simulink model "PickAndPlace_WithSelector"  (R2022b)
settings: Solver=ode4  StartTime=0.0  StopTime=Inf  FixedStep=1/500  RelTol=1e-3
InitFcn:
  | home = [0.45; 0; 0.49];
  | pick = [0.66; 0; 0.3];
  | place = [-0.425; 0.5; 0.35];
  | 
  | waypoints = ...
  | [pick, pick, place, place, home]' ;
undefined symbols (not defined in the file): HIL, pick2, place2, qc_get_step_size, waypoints2
libraries: quarc_library x5
settings Model: ExtModeTrigDuration=10000  Creator=fvranes  LastModifiedBy=user
settings SolverCC: AlgebraicLoopSolver=TrustRegion
settings DataIOCC: ReturnWorkspaceOutputs=off
settings DebuggingCC: UnderspecifiedInitializationDetection=Classic  MergeDetectMultiDrivingBlocksExec=none  UnconnectedInputMsg=warning  UnconnectedOutputMsg=warning  UnconnectedLineMsg=warning  SFMachineParentedDataDiag=warning
settings ModelReferenceCC: EnableRefExpFcnMdlSchedulingChecks=on  PropagateSignalLabelsOutOfModel=off
settings SFSimCC: CustomCodeUndefinedFunction=UseInterfaceOnly

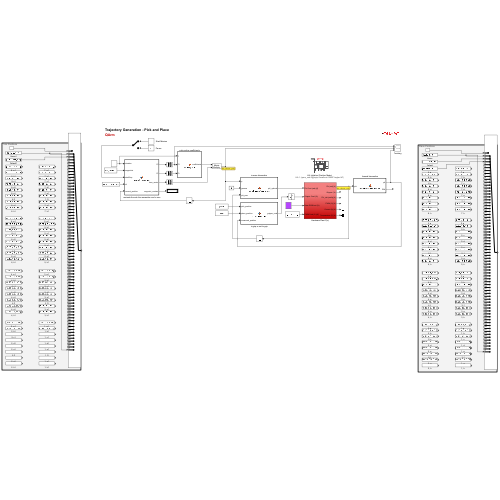
[thumbnail: Simulink's stored preview of the top-level diagram]
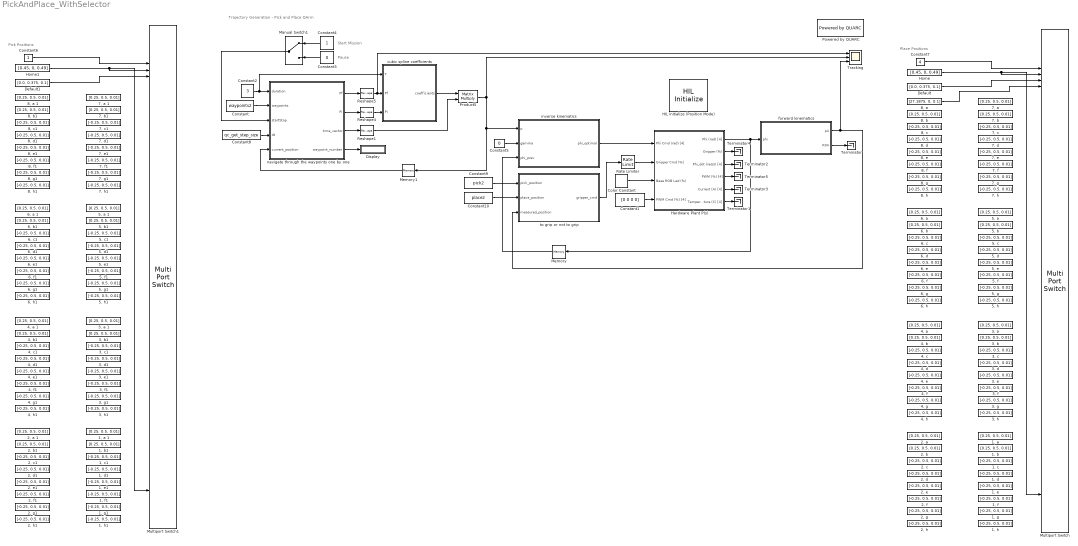
== system PickAndPlace_WithSelector ==
  note: Pause
  note: Start Mission
  note: Trajectory Generation - Pick and Place
      | QArm
  note: Place Positions
  note: Pick Positions
  "1, a " : Constant  Value=[0.25, 0.5, 0.01]
  "1, a 1" : Constant  Value=[0.25, 0.5, 0.01]
  "1, b" : Constant  Value=[0.25, 0.5, 0.01]
  "1, b1" : Constant  Value=[0.25, 0.5, 0.01]
  "1, c" : Constant  Value=[-0.25, 0.5, 0.01]
  "1, c1" : Constant  Value=[-0.25, 0.5, 0.01]
  "1, d" : Constant  Value=[-0.25, 0.5, 0.01]
  "1, d1" : Constant  Value=[-0.25, 0.5, 0.01]
  "1, e" : Constant  Value=[-0.25, 0.5, 0.01]
  "1, e1" : Constant  Value=[-0.25, 0.5, 0.01]
  "1, f" : Constant  Value=[-0.25, 0.5, 0.01]
  "1, f1" : Constant  Value=[-0.25, 0.5, 0.01]
  "1, g" : Constant  Value=[-0.25, 0.5, 0.01]
  "1, g1" : Constant  Value=[-0.25, 0.5, 0.01]
  "1, h" : Constant  Value=[-0.25, 0.5, 0.01]
  "1, h1" : Constant  Value=[-0.25, 0.5, 0.01]
  "2, a " : Constant  Value=[0.25, 0.5, 0.01]
  "2, a 1" : Constant  Value=[0.25, 0.5, 0.01]
  "2, b" : Constant  Value=[0.25, 0.5, 0.01]
  "2, b1" : Constant  Value=[0.25, 0.5, 0.01]
  "2, c" : Constant  Value=[-0.25, 0.5, 0.01]
  "2, c1" : Constant  Value=[-0.25, 0.5, 0.01]
  "2, d" : Constant  Value=[-0.25, 0.5, 0.01]
  "2, d1" : Constant  Value=[-0.25, 0.5, 0.01]
  "2, e" : Constant  Value=[-0.25, 0.5, 0.01]
  "2, e1" : Constant  Value=[-0.25, 0.5, 0.01]
  "2, f" : Constant  Value=[-0.25, 0.5, 0.01]
  "2, f1" : Constant  Value=[-0.25, 0.5, 0.01]
  "2, g" : Constant  Value=[-0.25, 0.5, 0.01]
  "2, g1" : Constant  Value=[-0.25, 0.5, 0.01]
  "2, h" : Constant  Value=[-0.25, 0.5, 0.01]
  "2, h1" : Constant  Value=[-0.25, 0.5, 0.01]
  "3, a " : Constant  Value=[0.25, 0.5, 0.01]
  "3, a 1" : Constant  Value=[0.25, 0.5, 0.01]
  "3, b" : Constant  Value=[0.25, 0.5, 0.01]
  "3, b1" : Constant  Value=[0.25, 0.5, 0.01]
  "3, c" : Constant  Value=[-0.25, 0.5, 0.01]
  "3, c1" : Constant  Value=[-0.25, 0.5, 0.01]
  "3, d" : Constant  Value=[-0.25, 0.5, 0.01]
  "3, d1" : Constant  Value=[-0.25, 0.5, 0.01]
  "3, e" : Constant  Value=[-0.25, 0.5, 0.01]
  "3, e1" : Constant  Value=[-0.25, 0.5, 0.01]
  "3, f" : Constant  Value=[-0.25, 0.5, 0.01]
  "3, f1" : Constant  Value=[-0.25, 0.5, 0.01]
  "3, g" : Constant  Value=[-0.25, 0.5, 0.01]
  "3, g1" : Constant  Value=[-0.25, 0.5, 0.01]
  "3, h" : Constant  Value=[-0.25, 0.5, 0.01]
  "3, h1" : Constant  Value=[-0.25, 0.5, 0.01]
  "4, a " : Constant  Value=[0.25, 0.5, 0.01]
  "4, a 1" : Constant  Value=[0.25, 0.5, 0.01]
  "4, b" : Constant  Value=[0.25, 0.5, 0.01]
  "4, b1" : Constant  Value=[0.25, 0.5, 0.01]
  "4, c" : Constant  Value=[-0.25, 0.5, 0.01]
  "4, c1" : Constant  Value=[-0.25, 0.5, 0.01]
  "4, d" : Constant  Value=[-0.25, 0.5, 0.01]
  "4, d1" : Constant  Value=[-0.25, 0.5, 0.01]
  "4, e" : Constant  Value=[-0.25, 0.5, 0.01]
  "4, e1" : Constant  Value=[-0.25, 0.5, 0.01]
  "4, f" : Constant  Value=[-0.25, 0.5, 0.01]
  "4, f1" : Constant  Value=[-0.25, 0.5, 0.01]
  "4, g" : Constant  Value=[-0.25, 0.5, 0.01]
  "4, g1" : Constant  Value=[-0.25, 0.5, 0.01]
  "4, h" : Constant  Value=[-0.25, 0.5, 0.01]
  "4, h1" : Constant  Value=[-0.25, 0.5, 0.01]
  "5, a " : Constant  Value=[0.25, 0.5, 0.01]
  "5, a 1" : Constant  Value=[0.25, 0.5, 0.01]
  "5, b" : Constant  Value=[0.25, 0.5, 0.01]
  "5, b1" : Constant  Value=[0.25, 0.5, 0.01]
  "5, c" : Constant  Value=[-0.25, 0.5, 0.01]
  "5, c1" : Constant  Value=[-0.25, 0.5, 0.01]
  "5, d" : Constant  Value=[-0.25, 0.5, 0.01]
  "5, d1" : Constant  Value=[-0.25, 0.5, 0.01]
  "5, e" : Constant  Value=[-0.25, 0.5, 0.01]
  "5, e1" : Constant  Value=[-0.25, 0.5, 0.01]
  "5, f" : Constant  Value=[-0.25, 0.5, 0.01]
  "5, f1" : Constant  Value=[-0.25, 0.5, 0.01]
  "5, g" : Constant  Value=[-0.25, 0.5, 0.01]
  "5, g1" : Constant  Value=[-0.25, 0.5, 0.01]
  "5, h" : Constant  Value=[-0.25, 0.5, 0.01]
  "5, h1" : Constant  Value=[-0.25, 0.5, 0.01]
  "6, a " : Constant  Value=[0.25, 0.5, 0.01]
  "6, a 1" : Constant  Value=[0.25, 0.5, 0.01]
  "6, b" : Constant  Value=[0.25, 0.5, 0.01]
  "6, b1" : Constant  Value=[0.25, 0.5, 0.01]
  "6, c" : Constant  Value=[-0.25, 0.5, 0.01]
  "6, c1" : Constant  Value=[-0.25, 0.5, 0.01]
  "6, d" : Constant  Value=[-0.25, 0.5, 0.01]
  "6, d1" : Constant  Value=[-0.25, 0.5, 0.01]
  "6, e" : Constant  Value=[-0.25, 0.5, 0.01]
  "6, e1" : Constant  Value=[-0.25, 0.5, 0.01]
  "6, f" : Constant  Value=[-0.25, 0.5, 0.01]
  "6, f1" : Constant  Value=[-0.25, 0.5, 0.01]
  "6, g" : Constant  Value=[-0.25, 0.5, 0.01]
  "6, g1" : Constant  Value=[-0.25, 0.5, 0.01]
  "6, h" : Constant  Value=[-0.25, 0.5, 0.01]
  "6, h1" : Constant  Value=[-0.25, 0.5, 0.01]
  "7, a " : Constant  Value=[0.25, 0.5, 0.01]
  "7, a 1" : Constant  Value=[0.25, 0.5, 0.01]
  "7, b" : Constant  Value=[0.25, 0.5, 0.01]
  "7, b1" : Constant  Value=[0.25, 0.5, 0.01]
  "7, c" : Constant  Value=[-0.25, 0.5, 0.01]
  "7, c1" : Constant  Value=[-0.25, 0.5, 0.01]
  "7, d" : Constant  Value=[-0.25, 0.5, 0.01]
  "7, d1" : Constant  Value=[-0.25, 0.5, 0.01]
  "7, e" : Constant  Value=[-0.25, 0.5, 0.01]
  "7, e1" : Constant  Value=[-0.25, 0.5, 0.01]
  "7, f" : Constant  Value=[-0.25, 0.5, 0.01]
  "7, f1" : Constant  Value=[-0.25, 0.5, 0.01]
  "7, g" : Constant  Value=[-0.25, 0.5, 0.01]
  "7, g1" : Constant  Value=[-0.25, 0.5, 0.01]
  "7, h" : Constant  Value=[-0.25, 0.5, 0.01]
  "7, h1" : Constant  Value=[-0.25, 0.5, 0.01]
  "8, a " : Constant  Value=[27.1875, 0, 0.1]
  "8, a 1" : Constant  Value=[0.25, 0.5, 0.01]
  "8, b" : Constant  Value=[0.25, 0.5, 0.01]
  "8, b1" : Constant  Value=[0.25, 0.5, 0.01]
  "8, c" : Constant  Value=[-0.25, 0.5, 0.01]
  "8, c1" : Constant  Value=[-0.25, 0.5, 0.01]
  "8, d" : Constant  Value=[-0.25, 0.5, 0.01]
  "8, d1" : Constant  Value=[-0.25, 0.5, 0.01]
  "8, e" : Constant  Value=[-0.25, 0.5, 0.01]
  "8, e1" : Constant  Value=[-0.25, 0.5, 0.01]
  "8, f" : Constant  Value=[-0.25, 0.5, 0.01]
  "8, f1" : Constant  Value=[-0.25, 0.5, 0.01]
  "8, g" : Constant  Value=[-0.25, 0.5, 0.01]
  "8, g1" : Constant  Value=[-0.25, 0.5, 0.01]
  "8, h" : Constant  Value=[-0.25, 0.5, 0.01]
  "8, h1" : Constant  Value=[-0.25, 0.5, 0.01]
  Color Constant : quarc_library/Sources/Signals/Color Constant  color=[0.71765 0.27451 1]
      settings: SourceProductName=QUARC Targets
  Constant : Constant  Value=waypoints2  VectorParams1D=off
  Constant1 : Constant  Value=[0 0 0 0]
  Constant10 : Constant  Value=place2  VectorParams1D=off
  Constant2 : Constant  Value=3
  Constant3 : Constant  Value=0
  Constant4 : Constant
  Constant5 : Constant  Value=0
  Constant6 : Constant
  Constant7 : Constant  Value=4
  Constant8 : Constant  Value=qc_get_step_size
  Constant9 : Constant  Value=pick2
  Default : Constant  Value=[0.0, 0.375, 0.1]
  Default1 : Constant  Value=[0.0, 0.375, 0.1]
  Display : Display
      settings: Decimation=2
  HIL Initialize (Position Mode) : quarc_library/Data Acquisition/Generic/Configuration/HIL Initialize  object_name=HIL-1  board_type=qarm_usb  board_number=0@tcpip://localhost:18900?nagle='off'  board_options=j0_mode=0;j1_mode=0;j2_mode=0;j3_mode=0;gripper_mode=0;  exclusive=off  active=on  hardware_clocks=[0]  clock_modes=[]  initial_clock_frequencies=[]  set_clock_params_at_start=off  set_clock_params_at_switch_in=off  set_clock_frequencies_at_start=off  set_clock_frequencies_at_switch_in=off  analog_input_channels=[5:9]  analog_input_configurations=[]  analog_input_maximums=[]  analog_input_minimums=[]  set_analog_input_params_at_start=off  set_analog_input_params_at_switch_in=off  analog_output_channels=[]  analog_output_maximums=inf  analog_output_minimums=-inf  initial_analog_outputs=[0]  final_analog_outputs=[0]  watchdog_analog_outputs=[]  set_analog_output_params_at_start=off  set_analog_output_params_at_switch_in=off  set_analog_outputs_at_start=off  set_analog_outputs_at_switch_in=off  set_analog_outputs_at_terminate=off  set_analog_outputs_at_switch_out=off  set_analog_outputs_on_watchdog=off  digital_input_channels=[]  digital_output_channels=[]  digital_output_configuration=[]  initial_digital_outputs=[0]  final_digital_outputs=[0]  watchdog_digital_outputs=[0]  set_digital_output_params_at_start=off  set_digital_output_params_at_switch_in=off  set_digital_outputs_at_start=off  set_digital_outputs_at_switch_in=off  set_digital_outputs_at_terminate=off  set_digital_outputs_at_switch_out=off  set_digital_outputs_on_watchdog=off  encoder_channels=[]  quadrature=[]  encoder_filter_frequency=[]  initial_encoder_counts=[]  set_encoder_params_at_start=off  set_encoder_params_at_switch_in=off  set_encoder_counts_at_start=off  set_encoder_counts_at_switch_in=off  pwm_channels=[]  pwm_modes=[]  pwm_frequency=[]  pwm_configuration=[]  pwm_alignment=[]  pwm_polarity=[]  pwm_leading_deadband=[]  pwm_trailing_deadband=[]  initial_pwm_outputs=[]  final_pwm_outputs=[]  watchdog_pwm_outputs=[]  set_pwm_params_at_start=off  set_pwm_params_at_switch_in=off  set_pwm_outputs_at_start=off  set_pwm_outputs_at_switch_in=off  set_pwm_outputs_at_terminate=off  set_pwm_outputs_at_switch_out=off  set_pwm_outputs_on_watchdog=off  other_output_channels=[1000:1004 11000:11003 11005:11007]  initial_other_outputs=[zeros(1,9), ones(1,3)]  final_other_outputs=[zeros(1,9), ones(1,3)]  watchdog_other_outputs=zeros(1,12)  set_other_outputs_at_start=off  set_other_outputs_at_switch_in=off  set_other_outputs_at_terminate=on  set_other_outputs_at_switch_out=off  set_other_outputs_on_watchdog=off
  Hardware Plant P(s) : Subsystem
  Home : Constant  Value=[0.45, 0, 0.49]
  Home1 : Constant  Value=[0.45, 0, 0.49]
  Manual Switch1 : ManualSwitch
  Memory : Memory
  Memory1 : Memory  InitialCondition=[0.45;0;0.49]
  Multiport Switch : MultiPortSwitch  Inputs=67  DataPortForDefault=Additional data port  SaturateOnIntegerOverflow=off  InputSameDT=off
  Multiport Switch1 : MultiPortSwitch  Inputs=67  DataPortForDefault=Additional data port  SaturateOnIntegerOverflow=off  InputSameDT=off
  Powered by QUARC : quarc_library/Logos/Powered by QUARC
  Product5 : Product  Multiplication=Matrix(*)
  Rate Limiter : RateLimiter  SampleTimeMode=inherited
  Reshape1 : Reshape  OutputDimensionality=Column vector (2-D)
  Reshape4 : Reshape  OutputDimensionality=Column vector (2-D)
  Reshape5 : Reshape  OutputDimensionality=Column vector (2-D)
  Terminator{,1..5} (6 alike) : Terminator
  Tracking : Scope  NumInputPorts=3
  cubic spline coefficients : MATLAB Function  TreatAsAtomicUnit=on
  forward kinematics : MATLAB Function  TreatAsAtomicUnit=on
  inverse kinematics : MATLAB Function  TreatAsAtomicUnit=on
  navigate through the waypoints one by one : MATLAB Function  TreatAsAtomicUnit=on
  to grip or not to grip : MATLAB Function  TreatAsAtomicUnit=on
  wires:
  Hardware Plant P(s)/4(PWM (%) [4]) -> Terminator5/1
  Hardware Plant P(s)/3(Phi_dot (rad/s) [4]) -> Terminator2/1
  Reshape1/1 -> Product5/2
  Hardware Plant P(s)/6(Temperature (C) [4]) -> Terminator1/1
  Memory1/1 -> navigate through the waypoints one by one/5(current_position)
  Memory/1 -> inverse kinematics/3(phi_prev)
  Rate Limiter/1 -> Hardware Plant P(s)/2(Gripper Cmd (%))
  Hardware Plant P(s)/5(Current (A) [4]) -> Terminator3/1
  Reshape4/1 -> cubic spline coefficients/3(Pi)
  Constant8/1 -> navigate through the waypoints one by one/4(dt)
  Color Constant/1 -> Hardware Plant P(s)/3(Base RGB Led (%))
  Constant3/1 -> Manual Switch1/2
  Constant1/1 -> Hardware Plant P(s)/4(PWM Cmd (%) [4])
  Manual Switch1/1 -> navigate through the waypoints one by one/3(startStop)
  Reshape5/1 -> Tracking/1, cubic spline coefficients/2(Pf)
  navigate through the waypoints one by one/4(waypoint_number) -> Display/1
  navigate through the waypoints one by one/1(Pf) -> Reshape5/1
  Hardware Plant P(s)/1(Phi (rad) [4]) -> forward kinematics/1(phi), Memory/1
  Constant5/1 -> inverse kinematics/2(gamma)
  Product5/1 -> Memory1/1, inverse kinematics/1(p), Tracking/2
  navigate through the waypoints one by one/2(Pi) -> Reshape4/1
  Constant4/1 -> Manual Switch1/1
  cubic spline coefficients/1(coefficients) -> Product5/1
  Constant2/1 -> cubic spline coefficients/1(T), navigate through the waypoints one by one/1(duration)
  forward kinematics/2(R04) -> Terminator/1
  forward kinematics/1(p4) -> Tracking/3, to grip or not to grip/3(measured_position)
  inverse kinematics/1(phi_optimal) -> Hardware Plant P(s)/1(Phi Cmd (rad) [4])
  to grip or not to grip/1(gripper_cmd) -> Rate Limiter/1
  navigate through the waypoints one by one/3(time_vector) -> Reshape1/1
  Hardware Plant P(s)/2(Gripper (%)) -> Terminator4/1
  Constant7/1 -> Multiport Switch/1
  Home/1 -> Multiport Switch/69, Multiport Switch/2
  Default/1 -> Multiport Switch/3
  Home1/1 -> Multiport Switch1/69, Multiport Switch1/2
  Constant6/1 -> Multiport Switch1/1
  Default1/1 -> Multiport Switch1/3
  "8, a "/1 -> Multiport Switch/4
  Constant10/1 -> to grip or not to grip/2(place_position)
  Constant9/1 -> to grip or not to grip/1(pick_position)
  Constant/1 -> navigate through the waypoints one by one/2(waypoints)

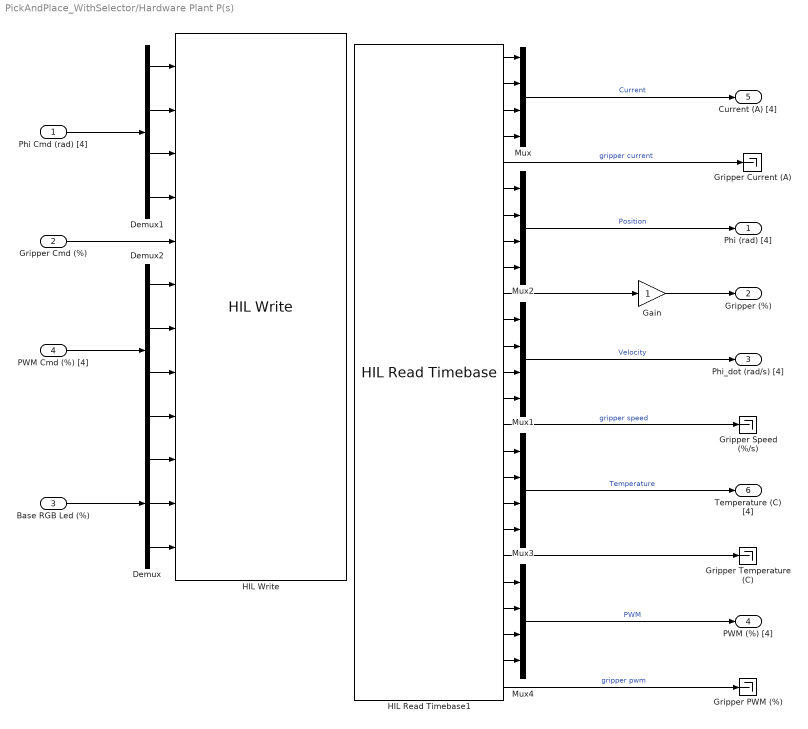
== system PickAndPlace_WithSelector/Hardware Plant P(s) ==
  Phi Cmd (rad) [4] : Inport
  Gripper Cmd (%) : Inport  Port=2
  Base RGB Led (%) : Inport  Port=3
  PWM Cmd (%) [4] : Inport  Port=4
  Demux : Demux  Outputs=3
  Demux1 : Demux
  Demux2 : Demux
  Gain : Gain
  Gripper Current (A) : Terminator
  Gripper PWM (%) : Terminator
  Gripper Speed (%/s) : Terminator
  Gripper Temperature (C) : Terminator
  HIL Read Timebase1 : quarc_library/Data Acquisition/Generic/Timebases/HIL Read Timebase  object_name=HIL-1  clock=0  analog_channels=[5:9]  encoder_channels=[]  digital_channels=[]  other_channels=[1000:1004 3000:3004 10000:10004 11000:11004]  active=on  vector_output=off  data_type_mode=Inherit via back propagation  encoder_data_type=double  digital_data_type=boolean  overflow_mode=Synchronize (for simulated cards only)  samples_in_buffer=1
  HIL Write : quarc_library/Data Acquisition/Generic/Immediate I//O/HIL Write  object_name=HIL-1  analog_channels=[]  pwm_channels=[]  digital_channels=[]  other_channels=[1000:1004 11000:11003 11005:11007]  sample_time=-1  active=on  vector_input=off
  Mux{,1..4} (5 alike) : Mux
  Phi (rad) [4] : Outport  VectorParamsAs1DForOutWhenUnconnected=off
  Gripper (%) : Outport  Port=2  VectorParamsAs1DForOutWhenUnconnected=off
  Phi_dot (rad/s) [4] : Outport  Port=3  VectorParamsAs1DForOutWhenUnconnected=off
  PWM (%) [4] : Outport  Port=4  VectorParamsAs1DForOutWhenUnconnected=off
  Current (A) [4] : Outport  Port=5  VectorParamsAs1DForOutWhenUnconnected=off
  Temperature (C) [4] : Outport  Port=6  VectorParamsAs1DForOutWhenUnconnected=off
  wires:
  HIL Read Timebase1/14 -> Mux1/4
  HIL Read Timebase1/9 -> Mux2/4
  HIL Read Timebase1/6 -> Mux2/1
  HIL Read Timebase1/18 -> Mux3/3
  HIL Read Timebase1/8 -> Mux2/3
  HIL Read Timebase1/12 -> Mux1/2
  HIL Read Timebase1/4 -> Mux/4
  HIL Read Timebase1/7 -> Mux2/2
  HIL Read Timebase1/5 -> Gripper Current (A)/1  "gripper current"
  HIL Read Timebase1/15 -> Gripper Speed (%/s)/1  "gripper speed"
  Demux/3 -> HIL Write/12
  HIL Read Timebase1/3 -> Mux/3
  HIL Read Timebase1/17 -> Mux3/2
  HIL Read Timebase1/16 -> Mux3/1
  HIL Read Timebase1/11 -> Mux1/1
  Demux/1 -> HIL Write/10
  HIL Read Timebase1/19 -> Mux3/4
  Demux/2 -> HIL Write/11
  HIL Read Timebase1/13 -> Mux1/3
  HIL Read Timebase1/2 -> Mux/2
  HIL Read Timebase1/1 -> Mux/1
  HIL Read Timebase1/20 -> Gripper Temperature (C)/1
  Mux/1 -> Current (A) [4]/1  "Current"
  Mux1/1 -> Phi_dot (rad/s) [4]/1  "Velocity"
  Mux3/1 -> Temperature (C) [4]/1  "Temperature"
  Base RGB Led (%)/1 -> Demux/1
  Demux1/1 -> HIL Write/1
  Demux1/2 -> HIL Write/2
  Demux1/3 -> HIL Write/3
  Demux1/4 -> HIL Write/4
  Phi Cmd (rad) [4]/1 -> Demux1/1
  PWM Cmd (%) [4]/1 -> Demux2/1
  Demux2/1 -> HIL Write/6
  Demux2/2 -> HIL Write/7
  Demux2/3 -> HIL Write/8
  Demux2/4 -> HIL Write/9
  Mux2/1 -> Phi (rad) [4]/1  "Position"
  HIL Read Timebase1/21 -> Mux4/1
  HIL Read Timebase1/22 -> Mux4/2
  HIL Read Timebase1/23 -> Mux4/3
  HIL Read Timebase1/24 -> Mux4/4
  HIL Read Timebase1/25 -> Gripper PWM (%)/1  "gripper pwm"
  Mux4/1 -> PWM (%) [4]/1  "PWM"
  HIL Read Timebase1/10 -> Gain/1
  Gain/1 -> Gripper (%)/1
  Gripper Cmd (%)/1 -> HIL Write/5

== matlab function PickAndPlace_WithSelector/navigate through the waypoints one by one ==
  data: duration input; waypoints input; Pf output; startStop input; dt input; current_position input; Pi output; time_vector output; waypoint_number output
function [Pf, Pi, time_vector, waypoint_number] = waypointNavigator(duration, waypoints, startStop, dt, current_position)

%% Initialization of internal variables
% Use persistent variables to track states across multiple iterations, and 
% define them on first call
persistent initial final next t
    if isempty(initial) || isempty(final)
        initial = current_position;
        final = current_position;
    end
    if isempty(next)
        next = 0;
    end
    if isempty(t)
        t = 0;
    end
    
% Find the number of waypoints in total    
[num_waypoints, ~] = size(waypoints);

%% Timing between the waypoints
% Ensure timer remains between 0 and duration
t_mod = mod(t, duration);

% Raise the flag if the timer resets to 0 (proceed to the next waypoint)
flag = t_mod < t;

%% Updating waypoints
if flag
    % proceed to the next waypoint
    next = next + 1;
    
    % cycle back to the first waypoint after the last one
    if next > num_waypoints
        next = 1;
    end

    % set the final and inital internal variables 
    final = waypoints(next, :)';
    initial = current_position;
end

%% Update the internal timer t
t = t_mod;
if startStop
    t = t + dt;
end

%% Set the outputs
waypoint_number = next; 
time_vector = [1; t; t^2; t^3];
Pf = final;
Pi = initial;

== matlab function PickAndPlace_WithSelector/cubic spline coefficients ==
  data: T input; coefficients output; Pf input; Pi input
function coefficients = cubicSpline(T, Pf, Pi)

% Cubic spline coefficients for X, Y and Z (coloumns)
a0 = [                     Pi(1,1);                      Pi(2,1);                     Pi(3,1)];
a1 = [                           0;                            0;                            0];
a2 = [ 3*(Pf(1,1) - Pi(1,1))/(T^2);  3*(Pf(2,1) - Pi(2,1))/(T^2);  3*(Pf(3,1) - Pi(3,1))/(T^2)];
a3 = [-2*(Pf(1,1) - Pi(1,1))/(T^3); -2*(Pf(2,1) - Pi(2,1))/(T^3); -2*(Pf(3,1) - Pi(3,1))/(T^3)];

% Output coefficients as a 3 x 4 matrix (1 row each for x, y and z)
coefficients = [a0, a1, a2, a3];

== matlab function PickAndPlace_WithSelector/forward kinematics ==
  data: phi input; p4 output; R04 output
function [p4, R04] = qarmForwardKinematics(phi)

%% QUANSER_ARM_FPK
% v 4.0 - 4th June 2020

% REFERENCE: 
% Chapter 3. Forward Kinematics
% Robot Dynamics and Control 
% Spong, Vidyasagar
% 1989

% INPUTS:
% phi     : Alternate joint angles vector 4 x 1

% OUTPUTS:
% p4      : End-effector frame {4} position vector expressed in base frame {0}
% R04     : rotation matrix from end-effector frame {4} to base frame {0}

%% Manipulator parameters:
L1 = 0.1400;
L2 = 0.3500;
L3 = 0.0500;
L4 = 0.2500;
L5 = 0.1500;

%% Alternate parameters
l1 = L1;
l2 = sqrt(L2^2 + L3^2);
l3 = L4 + L5;
beta = atan(L3/L2);

%% From phi space to theta space 
theta = phi;
theta(1) = phi(1);
theta(2) = phi(2) + beta - pi/2;
theta(3) = phi(3) - beta;
theta(4) = phi(4);

%% Transformation matrices for all frames:

% T{i-1}{i} = quanser_arm_DH(  a, alpha,  d,     theta );
        T01 = quanser_arm_DH(  0, -pi/2, l1,  theta(1) );
        T12 = quanser_arm_DH( l2,     0,  0,  theta(2) );
        T23 = quanser_arm_DH(  0, -pi/2,  0,  theta(3) );
        T34 = quanser_arm_DH(  0,     0, l3,  theta(4) );

        T02 = T01*T12;
        T03 = T02*T23;
        T04 = T03*T34;

%% Position of end-effector Transformation

% Extract the Position vector 
% p1   = T01(1:3,4);
% p2   = T02(1:3,4);
% p3   = T03(1:3,4);
p4   = T04(1:3,4);

% Extract the Rotation matrix
% R01 = T01(1:3,1:3);
% R02 = T02(1:3,1:3);
% R03 = T03(1:3,1:3);
R04 = T04(1:3,1:3);

end

function T = quanser_arm_DH(a,alpha,d,theta)

%% QUANSER_ARM_DH
% v 1.0 - 26th March 2019

% REFERENCE: 
% Chapter 3. Forward and Inverse Kinematics
% Robot Modeling and Control 
% Spong, Hutchinson, Vidyasagar
% 2006

% INPUTS:
% a       :   translation  : along : x_{i}   : from : z_{i-1} : to : z_{i}
% alpha   :      rotation  : about : x_{i}   : from : z_{i-1} : to : z_{i}
% d       :   translation  : along : z_{i-1} : from : x_{i-1} : to : x_{i}
% theta   :      rotation  : about : z_{i-1} : from : x_{i-1} : to : x_{i}
% NOTE: Standard DH Parameters

% OUTPUTS:
% T       : transformation                   : from :     {i} : to : {i-1}

%%
% Rotation Transformation about z axis by theta
T_R_z = [cos(theta) -sin(theta) 0 0;
         sin(theta)  cos(theta) 0 0;
                  0           0 1 0;
                  0           0 0 1];
     
% Translation Transformation along z axis by d
T_T_z = [1 0 0 0;
         0 1 0 0;
         0 0 1 d;
         0 0 0 1];

% Translation Transformation along x axis by a
T_T_x = [1 0 0 a;
         0 1 0 0;
         0 0 1 0;
         0 0 0 1];

% Rotation Transformation about x axis by alpha
T_R_x = [1          0           0 0;
         0 cos(alpha) -sin(alpha) 0;
         0 sin(alpha)  cos(alpha) 0;
         0          0           0 1];

% For a transformation FROM frame {i} TO frame {i-1}: A
T = T_R_z*T_T_z*T_T_x*T_R_x;

end

== matlab function PickAndPlace_WithSelector/inverse kinematics ==
  data: p input; gamma input; phi_optimal output; phi_prev input
function phi_optimal  = qarmInverseKinematics(p, gamma, phi_prev)

%% QUANSER_ARM_IPK
% v 4.0 - 4th June 2020

% REFERENCE: 
% Chapter 4. Inverse Kinematics
% Robot Dynamics and Control 
% Spong, Vidyasagar
% 1989

% INPUTS:
% p        : end-effector position vector expressed in base frame {0}
% gamma    : wrist rotation angle gamma

% OUTPUTS:
% phi_optimal : Best solution depending on phi_prev
% phi         : All four Inverse Kinematics solutions as a 4x4 matrix. 
%               Each col is a solution.

%% Manipulator parameters:
L1 = 0.1400;
L2 = 0.3500;
L3 = 0.0500;
L4 = 0.2500;
L5 = 0.1500;
beta = atan(L3/L2);

%% Alternate parameters
lambda1 = L1;
lambda2 = sqrt(L2^2 + L3^2);
lambda3 = L4 + L5;

%% Initialization
theta   = zeros(4, 4);
phi = zeros(4, 4);

%% Joint angle 2 and 3: 
% Equations:
    % lambda2 cos(theta2) + (-lambda3) sin(theta2 + theta3) = sqrt(x^2 + y^2)
    %   A     cos( 2    ) +     C      sin(   2   +    3  ) =    D
    
    % lambda2 sin(theta2) - (-lambda3) cos(theta2 + theta3) = lambda1 - z
    %   A     sin( 2    ) -     C      cos(   2   +    3  ) =    H

% Solution:
    A = lambda2;
    C = -lambda3;
    H =  lambda1 - p(3);
    D1 = -sqrt(p(1)^2 + p(2)^2);
    D2 = sqrt(p(1)^2 + p(2)^2);
    F = (D1^2 + H^2 - A^2 - C^2)/(2*A);

    theta(3,1) = 2*atan2( C + sqrt(C^2 - F^2) , F );
	theta(3,2) = 2*atan2( C - sqrt(C^2 - F^2) , F );
    theta(3,3) = 2*atan2( C + sqrt(C^2 - F^2) , F );
	theta(3,4) = 2*atan2( C - sqrt(C^2 - F^2) , F );

    M = A + C*sin(theta(3,1));
    N = -C*cos(theta(3,1));
    cos_term = (D1*M + H*N)/(M^2 + N^2);
    sin_term = (H - N*cos_term)/(M);
    theta(2,1) = atan2(sin_term, cos_term);

    M = A + C*sin(theta(3,2));
    N = -C*cos(theta(3,2));
    cos_term = (D1*M + H*N)/(M^2 + N^2);
    sin_term = (H - N*cos_term)/(M);
    theta(2,2) = atan2(sin_term, cos_term);

    M = A + C*sin(theta(3,3));
    N = -C*cos(theta(3,3));
    cos_term = (D2*M + H*N)/(M^2 + N^2);
    sin_term = (H - N*cos_term)/(M);
    theta(2,3) = atan2(sin_term, cos_term);

    M = A + C*sin(theta(3,4));
    N = -C*cos(theta(3,4));
    cos_term = (D2*M + H*N)/(M^2 + N^2);
    sin_term = (H - N*cos_term)/(M);
    theta(2,4) = atan2(sin_term, cos_term);


%% Joint angle 1:
% Equation:
    % y / x = tan(theta1);

% Solution
    theta(1,1) = atan2( p(2)/( lambda2 * cos( theta(2,1) ) - lambda3 * sin( theta(2,1) + theta(3,1) ) ) , p(1)/(  lambda2 * cos( theta(2,1) ) - lambda3 * sin( theta(2,1) + theta(3,1) )  ) );
    theta(1,2) = atan2( p(2)/( lambda2 * cos( theta(2,2) ) - lambda3 * sin( theta(2,2) + theta(3,2) ) ) , p(1)/(  lambda2 * cos( theta(2,2) ) - lambda3 * sin( theta(2,2) + theta(3,2) )  ) );
    theta(1,3) = atan2( p(2)/( lambda2 * cos( theta(2,3) ) - lambda3 * sin( theta(2,3) + theta(3,3) ) ) , p(1)/(  lambda2 * cos( theta(2,3) ) - lambda3 * sin( theta(2,3) + theta(3,3) )  ) );
    theta(1,4) = atan2( p(2)/( lambda2 * cos( theta(2,4) ) - lambda3 * sin( theta(2,4) + theta(3,4) ) ) , p(1)/(  lambda2 * cos( theta(2,4) ) - lambda3 * sin( theta(2,4) + theta(3,4) )  ) );
    
%% Remap theta back to phi
% phi(1) = theta(1);
% phi(2) = theta(2) - beta + pi/2;
% phi(3) = theta(3) + beta;
% phi(4) = theta(4);

phi(1,:) = theta(1,:);
phi(2,:) = theta(2,:) - beta + pi/2;
phi(3,:) = theta(3,:) + beta;
phi(4,:) = gamma;

phi = mod(phi + pi, 2*pi) - pi;

phi_optimal = phi(:,1);
if norm(phi_optimal - phi_prev) > norm(phi(:,2) - phi_prev)
    phi_optimal = phi(:,2);
end
if norm(phi_optimal - phi_prev) > norm(phi(:,3) - phi_prev)
    phi_optimal = phi(:,3);
end
if norm(phi_optimal - phi_prev) > norm(phi(:,4) - phi_prev)
    phi_optimal = phi(:,4);
end

end

== matlab function PickAndPlace_WithSelector/to grip or not to grip ==
  data: pick_position input; place_position input; measured_position input; gripper_cmd output
function gripper_cmd = actuateGripper(pick_position, place_position, measured_position)

% Define the internal gripper_state to be persistent and latch
persistent gripper_state
    if isempty(gripper_state)
        gripper_state = 0;
    end

% Actuate gripper if you are threshold meters away from destination
threshold = 0.03; % in meters

% If close to the pick position, close the gripper
if norm(pick_position - measured_position, 2) <= threshold && ~gripper_state
    gripper_state = 1;
end

% If close to the place position, open the gripper
if norm(place_position - measured_position, 2) <= threshold && gripper_state
    gripper_state = 0;
end

% Set the output to match the internal state
gripper_cmd = gripper_state;
